simulink model "EVdemo_6"  (R2013b)
settings: Solver=FixedStepDiscrete  SolverMode=SingleTasking  StartTime=0.0  StopTime=650  FixedStep=4e-5  MaxStep=1e-5  RelTol=1e-3
InitFcn:
  | %EV_Param_Update
  | % update the number of strings (discretized)
  | numStrings = round(Opti_numStrings);
  | %disp(['Number of strings: ' num2str(numStrings)])
  | % update the effective capacity based on the number of strings
  | EV_Param.Battery_Det.Rated_Capacity = 28.5*numStrings; %A*hr
  | EV_Param.Battery_Det.DP = 1.5*fliplr([1500 1500 1600 1450 1325 1125 925 675 425 175 ])./8*EV_Param.Battery_Det.Rated_Capacity; % 8 comes from the 8Ahr rated batter data used (normalize and rescale to the rated capacity
  | EV_Param.Battery_Det.CP = fliplr([25 100 200 250 375 550 750 950 1125 1150])./8*EV_Param.Battery_Det.Rated_Capacity;
  | 
  | % update the number of cells in a string (discretized)
  | numSeriesCells = round(Opti_numSeriesCells);
  | %disp(['Number of cells in a string: ' num2str(numSeriesCells)])
  | % update the nominal string volage and charge deficit
  | EV_Param.Battery_Det.Nominal_Voltage = numSeriesCells*cellVolts;
  | BatteryParams(1).Qe_init = 0;%EV_Param.Battery_Det.Rated_Capacity*(1-EV_Param.Battery_Det.Initial_SOC/100); %Ampere*hours
  | 
  | % update the total number of cells, battery pack mass and total vehicle
  | % mass
  | total_cells = numSeriesCells*numStrings;
  | %disp(['Total Number of cells: ' num2str(total_cells)])
  | EV_Param.BatteryMass = BatteryParams(1).cell_mass*total_cells;
  | %disp(['Total Battery Pack Mass: ' num2str(EV_Param.BatteryMass)])
  | EV_Param.Vehicle.Mass = 1300+EV_Param.BatteryMass;
  | 
  | % update the driveline gear ratio
  | EV_Param.Vehicle.Engine_Vehicle_Gear_Ratio = Opti_Vehicle_Gear_Ratio;
  | %disp(['Driveline gear ratio: ' num2str(Opti_Vehicle_Gear_Ratio)])
StartFcn:
  | %tic;
StopFcn:
  | %toc;
  | %disp([Final SOC: ' num2str(SOC_final)])
  | %disp([Final Vehicle Error: ' num2str(normed_SQE_final)])
model workspace (MAT data in the model file):
  MCOS : class17 (value not decoded)
  MCOS : class17 (value not decoded)
values from neighbouring files (symbols this model uses):
  Drive_Cycle_Num = 8    [startDemo.m]
undefined symbols (not defined in the file or in its folder): Acc_Cmd, BatteryParams, Brake_Set, cell_area, ctrlConst, current_phase_a, Dec_Cmd, direct_current, DiscIntNeverNeededParam, electromagnetic_torque, HEV_Param, Ion, Kt_Temps, Lithium, Mech_Power_kW, Opti_numSeriesCells, Opti_numStrings, Opti_Vehicle_Gear_Ratio, paramVelocityI, paramVelocityP, paramVelocityPICurrentSat, pmsm, quadrature_current, RLoadLoss, rotor_velocity, sigbuilder_block, Ts, Veh_Spd_Ref
libraries: fl_lib x306, nesl_utility x100, LeadAcidBattery_lib x60, simulink x23, powerlib x16, sdl_lib x7, elec_lib x4, electricdrivelib x2, checkpacklib x2, CustomDriveline_lib x2, LiBatteryBlocks x1, Capacitors_lib x1
(part 7 of 7)

== system EVdemo_6/Battery/RCGeneric/Measurements/Calculate battery power & charge ==
  -1/(60*60) : fl_lib/Physical Signals/Functions/PS Gain  gain=-1/(60*60)  LocalVarLogging=[]
  Initial charge Ah0 : Integrator  InitialCondition=HEV_Param.Battery_Sys.Maximum_Capacity
  PS Product : fl_lib/Physical Signals/Functions/PS Product  LocalVarLogging=[]
  PS Product1 : fl_lib/Physical Signals/Functions/PS Product  LocalVarLogging=[]
  PS-Simulink Converter : nesl_utility/PS-Simulink Converter  PhysicalDomain=network_engine_domain  SubClassName=ps_output  LeftPortType=input  RightPortType=output  PseudoPeriodic=off  Frequencies=[]  Unit=W  AffineConversion=off
  PS-Simulink Converter1 : nesl_utility/PS-Simulink Converter  PhysicalDomain=network_engine_domain  SubClassName=ps_output  LeftPortType=input  RightPortType=output  PseudoPeriodic=off  Frequencies=[]  Unit=1  AffineConversion=off
  PS-Simulink Converter2 : nesl_utility/PS-Simulink Converter  PhysicalDomain=network_engine_domain  SubClassName=ps_output  LeftPortType=input  RightPortType=output  PseudoPeriodic=off  Frequencies=[]  Unit=1  AffineConversion=off
  Rbat : Gain  Gain=HEV_Param.Battery_Sys.Internal_Resistance
  Terminator : Terminator
  Terminator1 : Terminator
  W to kW : Gain  Gain=1/1000
  V : PMIOPort  Port=1  Side=Left
  I : PMIOPort  Port=2  Side=Left
  Ah : Outport
  wires:
  PS-Simulink Converter/1 -> W to kW/1  "Battery power"
  W to kW/1 -> Terminator/1  "Pe_Batt"
  PS-Simulink Converter1/1 -> Initial charge Ah0/1  "d/dt(Ah)"
  Initial charge Ah0/1 -> Ah/1
  PS-Simulink Converter2/1 -> Rbat/1
  Rbat/1 -> Terminator1/1  "Pr_Batt"
  connections:
  PS Product/RConn1 -- PS-Simulink Converter/LConn1
  V/RConn1 -- PS Product/LConn1
  PS Product/LConn2 -- I/RConn1 -- -1/(60*60)/LConn1 -- PS Product1/LConn1 -- PS Product1/LConn2
  -1/(60*60)/RConn1 -- PS-Simulink Converter1/LConn1
  PS Product1/RConn1 -- PS-Simulink Converter2/LConn1

== system EVdemo_6/DCDC_Converter/Detailed DC//DC Converter/PWM/Sawtooth generator ==
  1\ib3 : Gain  Gain=2  SaturateOnIntegerOverflow=on  OutDataTypeStr=Inherit: Same as input  ParamDataTypeStr=Inherit: Same as input
  Constant1 : Constant  Value=20000
  Constant2 : Constant  Value=2
  Constant3 : Constant
  Discrete-Time Integrator : DiscreteIntegrator  IntegratorMethod=Integration: Trapezoidal  ExternalReset=rising  SampleTime=HEV_Param.DCDCConv.PWM_Carrier_TS  UpperSaturationLimit=1.5  LowerSaturationLimit=-1.5  ICPrevOutput=DiscIntNeverNeededParam  ICPrevScaledInput=DiscIntNeverNeededParam
  Relational Operator1 : RelationalOperator
  Sum1 : Sum  Inputs=+-  SaturateOnIntegerOverflow=on  InputSameDT=on  OutDataTypeStr=Inherit: Same as first input
  Unit Delay : UnitDelay  SampleTime=Ts
  Out : Outport
  wires:
  1\ib3/1 -> Discrete-Time Integrator/1
  Constant3/1 -> Sum1/2
  Sum1/1 -> Out/1
  Unit Delay/1 -> Discrete-Time Integrator/2
  Relational Operator1/1 -> Unit Delay/1
  Constant2/1 -> Relational Operator1/2
  Discrete-Time Integrator/1 -> Sum1/1, Relational Operator1/1
  Constant1/1 -> 1\ib3/1

== system EVdemo_6/DCDC_Converter/Detailed DC//DC Converter/PWM/Thermal Model ==
  IBus : Inport
  1/Mc : Gain  Gain=1/(HEV_Param.DCDCConv.Thermal_Mass*HEV_Param.DCDCConv.Specific_Heat)  SaturateOnIntegerOverflow=on  OutDataTypeStr=Inherit: Same as input  ParamDataTypeStr=Inherit: Same as input
  Air_Temp : Constant  Value=HEV_Param.DCDCConv.Air_Temperature-273
  Heat Losses : Gain  Gain=HEV_Param.DCDCConv.Convection.Area/HEV_Param.DCDCConv.Convection.HT_Coefficient  SaturateOnIntegerOverflow=on  OutDataTypeStr=Inherit: Same as input  ParamDataTypeStr=Inherit: Same as input
  Integrator : Integrator  InitialCondition=HEV_Param.DCDCConv.Initial_Temperature
  Subsystem : Subsystem
  Sum1 : Sum  Inputs=|+-  SaturateOnIntegerOverflow=on  InputSameDT=on  OutDataTypeStr=Inherit: Same as first input
  Sum2 : Sum  Inputs=|+-  SaturateOnIntegerOverflow=on  InputSameDT=on  OutDataTypeStr=Inherit: Same as first input
  tag scope: DCDC_SYS=global
  wires:
  Air_Temp/1 -> Sum2/2
  Subsystem/1(Heat Flow) -> Sum1/1  "Heat In"
  IBus/1 -> Subsystem/1(IBus)
  Integrator/1 -> Sum2/1, [DCDC_SYS]  "DCDC_Temp"
  1/Mc/1 -> Integrator/1
  Heat Losses/1 -> Sum1/2
  Sum2/1 -> Heat Losses/1
  Sum1/1 -> 1/Mc/1

== system EVdemo_6/DCDC_Converter/System DC-DC Converter/Control Bus Voltage/Bus_Control ==
  Err : Inport
  Add : Sum  OutMin=-ctrlConst.CurrentMax*2  OutMax=ctrlConst.CurrentMax*2  OutDataTypeStr=DT_PRECISION_HI  SaturateOnIntegerOverflow=on
      settings: AttributesFormatString=-----------------------------\nMin = %<OutMin>\nMax = %<OutMax>\nSat = %<SaturateOnIntegerOverflow>
  Clamp : Subsystem
  Constant : Constant  Value=0  OutDataTypeStr=Inherit: Inherit via back propagation  PreserveConstantTs=on
  Constant1 : Constant  Value=Ki  SampleTime=-1
  Constant2 : Constant  Value=EV_Param.DCDCConv.PWM_Carrier_TS  OutDataTypeStr=DT_PRECISION_LO  SampleTime=-1
  Convert_Data_Type : Subsystem
      mask Display: fprintf('Double\nRange')
  Maintain_Range : Subsystem
      mask Display: fprintf('Maintain\nRange')
  PI_Sat : Subsystem
      mask Display: plot([0.15 0.85],[.5 .5],[.5 .5],[0.05 0.95],0.15+0.7*[0 .25 .75 1],0.05+0.9*[.25 .25 .75 .75]);
  P_Gain : Gain  Gain=Kp  ParamDataTypeStr=Inherit: Inherit from 'Gain'
      settings: AttributesFormatString=-----------------------------\n%<Gain>
  Product : Product
  Product1 : Product
  Scope1 : Scope
      settings: SaveName=ScopeData13
  Scope2 : Scope
      settings: SaveName=ScopeData14
  Scope3 : Scope
      settings: SaveName=ScopeData15
  Sum : Sum  Inputs=++|
  Switch : Switch  Criteria=u2 > Threshold  InputSameDT=on
  Unit Delay : UnitDelay  SampleTime=-1
  V_Out : Outport
  wires:
  Maintain_Range/1(Out1) -> Product1/2
  Product/1 -> Maintain_Range/1(In1)
  Constant2/1 -> Product/2
  Constant1/1 -> Product/1
  Product1/1 -> Switch/3, Scope3/1, Clamp/3(preIntegrator)
  Clamp/1(Clamp) -> Switch/2
  Constant/1 -> Switch/1
  Unit Delay/1 -> Scope1/1, Sum/2, Add/2  "I_term"
  Add/1 -> Unit Delay/1
  P_Gain/1 -> Convert_Data_Type/1(In1)  "P_term"
  Err/1 -> P_Gain/1, Product1/1
  Switch/1 -> Add/1
  Convert_Data_Type/1(Out1) -> Sum/1, Scope2/1
  PI_Sat/2(saturated) -> Clamp/2(saturated)
  PI_Sat/1(Out1) -> V_Out/1
  Sum/1 -> PI_Sat/1(In1), Clamp/1(preSat)

== system EVdemo_6/Drive & Motor/Detailed_Motor/Motor And Sensors/PMSM_50kW ==
  note: Permanent Magnet
      | Synchronous Machine
  Group Signals : Subsystem
  Measures : electricdrivelib/AC drives/PM Synchronous Motor Drive/Measures
  Mechanical Rotational Reference : fl_lib/Mechanical/Rotational Elements/Mechanical Rotational Reference  t_Log=off  LocalVarNames=|t  LocalVarDescs=|t  LocalVarLogging=0
  Permanent Magnet Synchronous Machine : powerlib/Machines/Permanent Magnet Synchronous Machine  NbPhases=3  FluxDistribution=Sinusoidal  RotorType=Salient-pole  MechanicalLoad=Speed w  PresetModel=No  ShowDetailedParameters=on  Resistance=HEV_Param.Motor.Stator_Resistance  Inductance=8.5e-3  dqInductances=HEV_Param.Motor.Inductances  La=0.000835  MachineConstant=Flux linkage established by magnets (V.s)  Flux=0.175666143629361  VoltageCst=127.4493  TorqueCst=1.054  Flat=120  Mechanical=[0.00062 0.0003035 4 0]  PolePairs=4  InitialConditions=[0,0, 0,0]  InitialConditions5ph=[0 0 0 0 0 0]  TsPowergui=0  TsBlock=-1  RefAngle=Aligned with phase A axis (original Park)
  Rotational Damper : fl_lib/Mechanical/Rotational Elements/Rotational Damper  D=HEV_Param.Motor.Damping N*m/(rad/s)  t_Log=off  w_Log=off  LocalVarNames=|t|w  LocalVarDescs=|t|w  LocalVarLogging=[0 0]
  Shaft Inertia : fl_lib/Mechanical/Rotational Elements/Inertia  inertia=HEV_Param.Motor.Shaft_Inertia kg*m^2  initial_velocity=0 rad/s  t_Log=off  LocalVarNames=|t  LocalVarDescs=|t  LocalVarLogging=0
  Subsystem : Subsystem
      mask Display: disp('GF');
  Subsystem1 : Subsystem
  Terminator : Terminator
  R : PMIOPort  Port=1  Side=Right
  A : PMIOPort  Port=2  Side=Left
  B : PMIOPort  Port=3  Side=Left
  C : PMIOPort  Port=4  Side=Left
  M : Outport
  wires:
  Measures/1 -> Terminator/1
  Permanent Magnet Synchronous Machine/1 -> Subsystem/1(In), Group Signals/1(M)
  Subsystem/1(Out) -> Subsystem1/1(Sig)
  Subsystem1/1(Spd) -> Permanent Magnet Synchronous Machine/1
  Group Signals/1(O) -> M/1  "motor"
  connections:
  C/RConn1 -- Measures/LConn3
  B/RConn1 -- Measures/LConn2
  A/RConn1 -- Measures/LConn1
  Permanent Magnet Synchronous Machine/LConn3 -- Measures/RConn3
  R/RConn1 -- Rotational Damper/LConn1 -- Subsystem1/RConn1 -- Shaft Inertia/LConn1
  Permanent Magnet Synchronous Machine/LConn1 -- Measures/RConn1
  Permanent Magnet Synchronous Machine/LConn2 -- Measures/RConn2
  Mechanical Rotational Reference/LConn1 -- Rotational Damper/RConn1

== system EVdemo_6/Drive & Motor/Detailed_Motor/Motor And Sensors/Temperature Sensor ==
  Ideal Temperature Sensor : fl_lib/Thermal/Thermal Sensors/Ideal Temperature Sensor  Qs_Log=off  Ts_Log=off  LocalVarNames=|Qs|Ts  LocalVarDescs=|Qs|Ts  LocalVarLogging=[]
  PS-Simulink Converter : nesl_utility/PS-Simulink Converter  PhysicalDomain=network_engine_domain  SubClassName=ps_output  LeftPortType=input  RightPortType=output  PseudoPeriodic=off  Frequencies=[]  Unit=C  AffineConversion=on
  Rate Transition5 : RateTransition  OutPortSampleTime=.01
  Thermal Reference : fl_lib/Thermal/Thermal Elements/Thermal Reference  Q_Log=off  LocalVarNames=|Q  LocalVarDescs=|Q  LocalVarLogging=[]
  Conn2 : PMIOPort  Port=1  Side=Left
  tag scope: DCDC_SYS=global
  wires:
  PS-Simulink Converter/1 -> Rate Transition5/1  "DCDC_Temp"
  Rate Transition5/1 -> [DCDC_SYS]
  connections:
  Conn2/RConn1 -- Ideal Temperature Sensor/LConn1
  Thermal Reference/LConn1 -- Ideal Temperature Sensor/RConn1
  PS-Simulink Converter/LConn1 -- Ideal Temperature Sensor/RConn2

== system EVdemo_6/Drive & Motor/System_Motor/Control_Velocity (Explicit_Ts)/Rotor_Velocity_Control ==
  Err : Inport
  mtr_torque_lim : Inport  Port=2  OutMin=-ctrlConst.VelocityMax  OutMax=ctrlConst.VelocityMax
  regen_torque_lim : Inport  Port=3  OutMin=-ctrlConst.VelocityMax  OutMax=ctrlConst.VelocityMax
  Add : Sum  OutMin=-ctrlConst.CurrentMax*2  OutMax=ctrlConst.CurrentMax*2  OutDataTypeStr=DT_PRECISION_HI  SaturateOnIntegerOverflow=on
      settings: AttributesFormatString=-----------------------------\nMin = %<OutMin>\nMax = %<OutMax>\nSat = %<SaturateOnIntegerOverflow>
  Clamp : Subsystem
  Constant : Constant  Value=0  OutDataTypeStr=Inherit: Inherit via back propagation  PreserveConstantTs=on
  Constant1 : Constant  Value=paramVelocityI  SampleTime=-1
  Constant2 : Constant  Value=ctrlConst.Ts  OutDataTypeStr=DT_PRECISION_LO  SampleTime=-1
  Convert_Data_Type : Subsystem
      mask Display: fprintf('Double\nRange')
  Data Type Conversion1 : DataTypeConversion  OutMin=-ctrlConst.CurrentMax  OutMax=ctrlConst.CurrentMax  OutDataTypeStr=DT_PRECISION_LO
      settings: AttributesFormatString=-----------------------------\nMin = %<OutMin>\nMax = %<OutMax>
  Dynamic Saturation : Subsystem
      mask Display: plot([0.15 0.85],[.5 .5],[.5 .5],[0.05 0.95],0.15+0.7*[0 .25 .75 1],0.05+0.9*[.25 .25 .75 .75]);
  Maintain_Range : Subsystem
      mask Display: fprintf('Maintain\nRange')
  PI_Sat1 : Constant  Commented=on  Value=paramVelocityPICurrentSat  PreserveConstantTs=on
  P_Gain : Gain  Gain=paramVelocityP  ParamDataTypeStr=Inherit: Inherit from 'Gain'
      settings: AttributesFormatString=-----------------------------\n%<Gain>
  Product : Product
  Product1 : Product
  Sum : Sum  Inputs=++|
  Switch : Switch  Criteria=u2 > Threshold  InputSameDT=on
  Unit Delay : UnitDelay  SampleTime=-1
  Out : Outport
  wires:
  Data Type Conversion1/1 -> Out/1
  Dynamic Saturation/1(y) -> Data Type Conversion1/1
  Maintain_Range/1(Out1) -> Product1/2
  Product/1 -> Maintain_Range/1(In1)
  Constant2/1 -> Product/2
  Constant1/1 -> Product/1
  Product1/1 -> Switch/3, Clamp/3(preIntegrator)
  Clamp/1(Clamp) -> Switch/2
  Constant/1 -> Switch/1
  Unit Delay/1 -> Sum/2, Add/2  "I_term"
  Add/1 -> Unit Delay/1
  P_Gain/1 -> Convert_Data_Type/1(In1)  "P_term"
  Sum/1 -> Dynamic Saturation/2(u), Clamp/1(preSat)
  Err/1 -> P_Gain/1, Product1/1
  Dynamic Saturation/2(sat_mode) -> Clamp/2(saturated)
  Switch/1 -> Add/1
  Convert_Data_Type/1(Out1) -> Sum/1
  mtr_torque_lim/1 -> Dynamic Saturation/1(up)
  regen_torque_lim/1 -> Dynamic Saturation/3(lo)

== system EVdemo_6/Drive & Motor/System_Motor/Synchronous Motor & Drive/Calculate electrical power ==
  Current Sensor : fl_lib/Electrical/Electrical Sensors/Current Sensor  i1_Log=off  v1_Log=off  LocalVarNames=|i1|v1  LocalVarDescs=|i1|v1  LocalVarLogging=[]
  PS Product1 : fl_lib/Physical Signals/Functions/PS Product  LocalVarLogging=[]
  PS-Simulink Converter : nesl_utility/PS-Simulink Converter  PhysicalDomain=network_engine_domain  SubClassName=ps_output  LeftPortType=input  RightPortType=output  PseudoPeriodic=off  Frequencies=[]  Unit=1  AffineConversion=off
  PS-Simulink Converter1 : nesl_utility/PS-Simulink Converter  PhysicalDomain=network_engine_domain  SubClassName=ps_output  LeftPortType=input  RightPortType=output  PseudoPeriodic=off  Frequencies=[]  Unit=1  AffineConversion=off
  PS-Simulink Converter4 : nesl_utility/PS-Simulink Converter  PhysicalDomain=network_engine_domain  SubClassName=ps_output  LeftPortType=input  RightPortType=output  PseudoPeriodic=off  Frequencies=[]  Unit=1  AffineConversion=off
  Voltage Sensor : fl_lib/Electrical/Electrical Sensors/Voltage Sensor  i1_Log=off  v1_Log=off  LocalVarNames=|i1|v1  LocalVarDescs=|i1|v1  LocalVarLogging=[]
  W to kW : Gain  Gain=1/1000
  + : PMIOPort  Port=1  Side=Left
  ref : PMIOPort  Port=2  Side=Left
  - : PMIOPort  Port=3  Side=Right
  tag scope: Drive_Bus_Current=global, Drive_Bus_Voltage=global, Drive_DC_Power_kW=global
  wires:
  PS-Simulink Converter1/1 -> [Drive_Bus_Current]
  PS-Simulink Converter/1 -> [Drive_Bus_Voltage]
  PS-Simulink Converter4/1 -> W to kW/1
  W to kW/1 -> [Drive_DC_Power_kW]
  connections:
  ref/RConn1 -- Voltage Sensor/RConn2
  +/RConn1 -- Current Sensor/LConn1
  PS-Simulink Converter4/LConn1 -- PS Product1/RConn1
  PS-Simulink Converter/LConn1 -- PS Product1/LConn2 -- Voltage Sensor/RConn1
  Voltage Sensor/LConn1 -- Current Sensor/RConn2 -- -/RConn1
  PS Product1/LConn1 -- PS-Simulink Converter1/LConn1 -- Current Sensor/RConn1

== system EVdemo_6/Drive & Motor/System_Motor/Synchronous Motor & Drive/Calculate mechanical power ==
  Ideal Rotational Motion Sensor : fl_lib/Mechanical/Mechanical Sensors/Ideal Rotational Motion Sensor  offset=0 rad  w_Log=off  t_Log=off  phi_Log=off  LocalVarNames=|w|t|phi  LocalVarDescs=|w|t|phi  LocalVarLogging=[]
  Mechanical Rotational Reference1 : fl_lib/Mechanical/Rotational Elements/Mechanical Rotational Reference  t_Log=off  LocalVarNames=|t  LocalVarDescs=|t  LocalVarLogging=[]
  PS Product : fl_lib/Physical Signals/Functions/PS Product  LocalVarLogging=[]
  PS-Simulink Converter1 : nesl_utility/PS-Simulink Converter  PhysicalDomain=network_engine_domain  SubClassName=ps_output  LeftPortType=input  RightPortType=output  PseudoPeriodic=off  Frequencies=[]  Unit=N*m  AffineConversion=off
  PS-Simulink Converter2 : nesl_utility/PS-Simulink Converter  PhysicalDomain=network_engine_domain  SubClassName=ps_output  LeftPortType=input  RightPortType=output  PseudoPeriodic=off  Frequencies=[]  Unit=rad/s  AffineConversion=off
  PS-Simulink Converter3 : nesl_utility/PS-Simulink Converter  PhysicalDomain=network_engine_domain  SubClassName=ps_output  LeftPortType=input  RightPortType=output  PseudoPeriodic=off  Frequencies=[]  Unit=1  AffineConversion=off
  Torque Sensor : fl_lib/Mechanical/Mechanical Sensors/Ideal Torque Sensor  w_Log=off  t_Log=off  LocalVarNames=|w|t  LocalVarDescs=|w|t  LocalVarLogging=[]
  W to kW : Gain  Gain=1/1000
  C : PMIOPort  Port=1  Side=Right
  R : PMIOPort  Port=2  Side=Left
  tag scope: Motor_Mech_Power_kW=global, Motor_Speed_radps=global, Motor_Torque_Nm=global
  wires:
  PS-Simulink Converter2/1 -> [Motor_Speed_radps]
  W to kW/1 -> [Motor_Mech_Power_kW]
  PS-Simulink Converter3/1 -> W to kW/1
  PS-Simulink Converter1/1 -> [Motor_Torque_Nm]
  connections:
  Mechanical Rotational Reference1/LConn1 -- Ideal Rotational Motion Sensor/RConn1
  PS Product/LConn2 -- PS-Simulink Converter2/LConn1 -- Ideal Rotational Motion Sensor/RConn2
  Torque Sensor/RConn2 -- PS-Simulink Converter1/LConn1 -- PS Product/LConn1
  PS Product/RConn1 -- PS-Simulink Converter3/LConn1
  Ideal Rotational Motion Sensor/LConn1 -- Torque Sensor/LConn1 -- R/RConn1
  C/RConn1 -- Torque Sensor/RConn1

== system EVdemo_6/Drive & Motor/System_Motor/Synchronous Motor & Drive/GF ==
  In1 : Inport
  Simulink-PS Converter : nesl_utility/Simulink-PS Converter  PhysicalDomain=network_engine_domain  SubClassName=ps_input  LeftPortType=input  RightPortType=output  PseudoPeriodic=off  Frequencies=[]  NoiseDistribution=none  NoiseParameters=[]  Unit=1  AffineConversion=off  InputFiltering=off  SimscapeFilterOrder=1  InputFilterTimeConstant=.001  UdotUserProvided=0
  Conn1 : PMIOPort  Port=1  Side=Right
  tag scope: Motor_Torque_Ref=global
  wires:
  In1/1 -> Simulink-PS Converter/1, [Motor_Torque_Ref]
  connections:
  Simulink-PS Converter/RConn1 -- Conn1/RConn1

== system EVdemo_6/Drive & Motor/System_Motor/Synchronous Motor & Drive/PS Terminator1 ==
  PS-Simulink Converter 2 : nesl_utility/PS-Simulink Converter  PhysicalDomain=network_engine_domain  SubClassName=ps_output  LeftPortType=input  RightPortType=output  PseudoPeriodic=off  Frequencies=[]  Unit=rpm  AffineConversion=off
  Terminator : Terminator
  R : PMIOPort  Port=1  Side=Left
  wires:
  PS-Simulink Converter 2/1 -> Terminator/1
  connections:
  R/RConn1 -- PS-Simulink Converter 2/LConn1

== system EVdemo_6/Operator Model/Accel_Cmd_Gen/PI_Sat/Dynamic Saturation ==
  up : Inport
  u : Inport  Port=2
  lo : Inport  Port=3
  Logical Operator : Logic  Operator=OR  AllPortsSameDT=off  OutDataTypeStr=boolean
  LowerRelop1 : RelationalOperator  DisableCoverage=on  Operator=>  OutDataTypeStr=boolean
  Switch : Switch  Criteria=u2 ~= 0  ZeroCross=off
  Switch2 : Switch  Criteria=u2 ~= 0  ZeroCross=off
  UpperRelop : RelationalOperator  DisableCoverage=on  Operator=<  OutDataTypeStr=boolean
  y : Outport
  sat_mode : Outport  Port=2
  wires:
  Logical Operator/1 -> sat_mode/1
  up/1 -> Switch2/1, LowerRelop1/2
  u/1 -> LowerRelop1/1, Switch/3, UpperRelop/1
  lo/1 -> Switch/1, UpperRelop/2
  Switch/1 -> Switch2/3
  Switch2/1 -> y/1
  LowerRelop1/1 -> Switch2/2, Logical Operator/1
  UpperRelop/1 -> Switch/2, Logical Operator/2

== system EVdemo_6/Operator Model/Brake_Cmd_Gen/PI_Sat/Dynamic Saturation ==
  up : Inport
  u : Inport  Port=2
  lo : Inport  Port=3
  Logical Operator : Logic  Operator=OR  AllPortsSameDT=off  OutDataTypeStr=boolean
  LowerRelop1 : RelationalOperator  DisableCoverage=on  Operator=>  OutDataTypeStr=boolean
  Switch : Switch  Criteria=u2 ~= 0  ZeroCross=off
  Switch2 : Switch  Criteria=u2 ~= 0  ZeroCross=off
  UpperRelop : RelationalOperator  DisableCoverage=on  Operator=<  OutDataTypeStr=boolean
  y : Outport
  sat_mode : Outport  Port=2
  wires:
  UpperRelop/1 -> Logical Operator/2, Switch/2
  LowerRelop1/1 -> Logical Operator/1, Switch2/2
  Switch2/1 -> y/1
  Switch/1 -> Switch2/3
  lo/1 -> UpperRelop/2, Switch/1
  u/1 -> UpperRelop/1, Switch/3, LowerRelop1/1
  up/1 -> LowerRelop1/2, Switch2/1
  Logical Operator/1 -> sat_mode/1

== system EVdemo_6/DCDC_Converter/Detailed DC//DC Converter/PWM/Thermal Model/Subsystem ==
  IBus : Inport
  PToHeat : Gain  Gain=HEV_Param.DCDCConv.EPower2Heat  SaturateOnIntegerOverflow=on  OutDataTypeStr=Inherit: Same as input  ParamDataTypeStr=Inherit: Same as input
  Product : Product  RndMeth=Zero
  RLoss : Gain  Gain=HEV_Param.DCDCConv.Resistance_Losses  SaturateOnIntegerOverflow=on  OutDataTypeStr=Inherit: Same as input  ParamDataTypeStr=Inherit: Same as input
  Heat Flow : Outport
  wires:
  PToHeat/1 -> Heat Flow/1
  RLoss/1 -> PToHeat/1
  IBus/1 -> Product/2, Product/1
  Product/1 -> RLoss/1

== system EVdemo_6/DCDC_Converter/System DC-DC Converter/Control Bus Voltage/Bus_Control/Clamp ==
  preSat : Inport
  saturated : Inport  Port=2
  preIntegrator : Inport  Port=3
  AND : Logic  OutDataTypeStr=boolean
  Compare To Zero : simulink/Logic and Bit Operations/Compare To Zero  relop=<=  OutDataTypeStr=boolean
  Compare To Zero1 : simulink/Logic and Bit Operations/Compare To Zero  relop=<=  OutDataTypeStr=boolean
  Logical Operator : Logic  Operator=NXOR  AllPortsSameDT=off  OutDataTypeStr=boolean
  Clamp : Outport
  wires:
  Compare To Zero1/1 -> Logical Operator/2
  Compare To Zero/1 -> Logical Operator/1
  Logical Operator/1 -> AND/1
  preSat/1 -> Compare To Zero1/1
  preIntegrator/1 -> Compare To Zero/1
  saturated/1 -> AND/2
  AND/1 -> Clamp/1

== system EVdemo_6/DCDC_Converter/System DC-DC Converter/Control Bus Voltage/Bus_Control/Convert_Data_Type ==
  In1 : Inport
  Data Type Conversion : DataTypeConversion  Priority=27
  Data Type Propagation : simulink/Signal Attributes/Data Type Propagation  Priority=24  PropDataType=fixdt(1, 16)  IfRefDouble=double  IfRefSingle=single  IsSigned=IsSigned1  NumBitsBase=NumBits1  NumBitsMult=1  NumBitsAdd=0  NumBitsAllowFinal=1:128  PropScaling=2^-10  ValuesUsedBestPrec=[5 -7]  SlopeBase=Slope1  SlopeMult=2  SlopeAdd=0  BiasBase=Bias1  BiasMult=1  BiasAdd=0
      settings: AttributesFormatString=-------------------------------\nDT = %<PropDataType>
  Out1 : Outport
  wires:
  Data Type Conversion/1 -> Data Type Propagation/3, Out1/1
  In1/1 -> Data Type Conversion/1, Data Type Propagation/1, Data Type Propagation/2

== system EVdemo_6/DCDC_Converter/System DC-DC Converter/Control Bus Voltage/Bus_Control/Maintain_Range ==
  In1 : Inport
  Data Type Conversion : DataTypeConversion
  Data Type Propagation : simulink/Signal Attributes/Data Type Propagation  PropDataTypeMode=Specify via dialog  PropDataType=DT_PRECISION_LO  IfRefDouble=double  IfRefSingle=single  IsSigned=IsSigned1  NumBitsBase=NumBits1  NumBitsMult=0  NumBitsAdd=0  NumBitsAllowFinal=1:128  PropScaling=2^-10  ValuesUsedBestPrec=[5 -7]  SlopeBase=PosRange1  SlopeMult=1  SlopeAdd=0  BiasBase=Bias1  BiasMult=1  BiasAdd=0
      settings: AttributesFormatString=-------------------------------\nDT = %<PropDataType>
  Out1 : Outport
  wires:
  Data Type Conversion/1 -> Data Type Propagation/3, Out1/1
  In1/1 -> Data Type Conversion/1, Data Type Propagation/1, Data Type Propagation/2

== system EVdemo_6/DCDC_Converter/System DC-DC Converter/Control Bus Voltage/Bus_Control/PI_Sat ==
  In1 : Inport
  Dynamic Saturation : Subsystem
      mask Display: plot([0.15 0.85],[.5 .5],[.5 .5],[0.05 0.95],0.15+0.7*[0 .25 .75 1],0.05+0.9*[.25 .25 .75 .75]);
  PI_Sat : Constant  Value=800  PreserveConstantTs=on
  PI_Sat1 : Constant  Value=12  PreserveConstantTs=on
  Out1 : Outport
  saturated : Outport  Port=2
  wires:
  In1/1 -> Dynamic Saturation/2(u)
  PI_Sat/1 -> Dynamic Saturation/1(up)
  PI_Sat1/1 -> Dynamic Saturation/3(lo)
  Dynamic Saturation/1(y) -> Out1/1
  Dynamic Saturation/2(sat_mode) -> saturated/1

== system EVdemo_6/Drive & Motor/Detailed_Motor/Motor And Sensors/PMSM_50kW/Group Signals ==
  note: Group Signals
  note: Rename signals provided to output bus.
  M : Inport
  Bus Creator2 : BusCreator  Inputs=10
  Bus Selector2 : BusSelector  OutputSignals=Stator current is_a (A),Stator current is_b (A),Stator current is_c (A),Electromagnetic torque Te (N*m),Rotor speed wm (rad/s),Stator current is_d (A),Stator current is_q (A),Rotor angle thetam (rad)
  Mechanical To Electrical : Subsystem
  Signal Conversion {1..5,7..8} (7 alike) : SignalConversion  ConversionOutput=Contiguous copy
  Wrap 2pi : Subsystem
  O : Outport
  wires:
  Bus Creator2/1 -> O/1  "measure"
  M/1 -> Bus Selector2/1, Mechanical To Electrical/1(M)
  Bus Selector2/1 -> Signal Conversion 1/1  "<Stator current is_a (A)>"
  Bus Selector2/2 -> Signal Conversion 2/1  "<Stator current is_b (A)>"
  Bus Selector2/3 -> Signal Conversion 3/1  "<Stator current is_c (A)>"
  Bus Selector2/5 -> Signal Conversion 5/1  "<Rotor speed wm (rad/s)>"
  Bus Selector2/4 -> Signal Conversion 4/1  "<Electromagnetic torque Te (N*m)>"
  Signal Conversion 1/1 -> Bus Creator2/1  "current_phase_a"
  Signal Conversion 2/1 -> Bus Creator2/2  "current_phase_b"
  Signal Conversion 3/1 -> Bus Creator2/3  "current_phase_c"
  Signal Conversion 4/1 -> Bus Creator2/4  "electromagnetic_torque"
  Signal Conversion 5/1 -> Bus Creator2/5  "rotor_velocity"
  Bus Selector2/8 -> Wrap 2pi/1(M)  "<Rotor angle thetam (rad)>"
  Signal Conversion 7/1 -> Bus Creator2/6  "direct_current"
  Signal Conversion 8/1 -> Bus Creator2/7  "quadrature_current"
  Bus Selector2/6 -> Signal Conversion 7/1  "<Stator current is_d (A)>"
  Bus Selector2/7 -> Signal Conversion 8/1  "<Stator current is_q (A)>"
  Wrap 2pi/1(Position) -> Bus Creator2/8  "rotor_position"
  Mechanical To Electrical/1(Position) -> Bus Creator2/9  "electrical_position"
  Mechanical To Electrical/2(Velocity) -> Bus Creator2/10  "electrical_velocity"

== system EVdemo_6/Drive & Motor/Detailed_Motor/Motor And Sensors/PMSM_50kW/Subsystem ==
  In : Inport
  "+ -> -1" : Gain  Gain=30/pi
  Bus Selector : BusSelector  OutputSignals=Stator current is_a (A),Rotor speed wm (rad/s),Electromagnetic torque Te (N*m)
  Mux1 : Mux  Inputs=2
  Mux2 : Mux  Inputs=3
  Out : Outport
  tag scope: MotorDrive=global
  wires:
  In/1 -> Bus Selector/1, Out/1
  "+ -> -1"/1 -> Mux2/2
  [Mot_TReq_SYS] -> Mux1/2
  Bus Selector/2 -> "+ -> -1"/1  "<Rotor speed wm (rad/s)>"
  Bus Selector/3 -> Mux1/1  "<Electromagnetic torque Te (N*m)>"
  Mux1/1 -> Mux2/3
  Bus Selector/1 -> Mux2/1  "<Stator current is_a (A)>"
  Mux2/1 -> [MotorDrive]

== system EVdemo_6/Drive & Motor/Detailed_Motor/Motor And Sensors/PMSM_50kW/Subsystem1 ==
  Sig : Inport
  Bus Selector : BusSelector  OutputSignals=Electromagnetic torque Te (N*m)
  Ideal Rotational Motion Sensor : fl_lib/Mechanical/Mechanical Sensors/Ideal Rotational Motion Sensor  offset=0 rad  w_Log=off  t_Log=off  phi_Log=off  LocalVarNames=|w|t|phi  LocalVarDescs=|w|t|phi  LocalVarLogging=[0 0 0]
  Ideal Torque Source : fl_lib/Mechanical/Mechanical Sources/Ideal Torque Source  w_Log=off  t_Log=off  LocalVarNames=|w|t  LocalVarDescs=|w|t  LocalVarLogging=[0 0]
  Mechanical Rotational Reference : fl_lib/Mechanical/Rotational Elements/Mechanical Rotational Reference  t_Log=off  LocalVarNames=|t  LocalVarDescs=|t  LocalVarLogging=0
  Mechanical Rotational Reference1 : fl_lib/Mechanical/Rotational Elements/Mechanical Rotational Reference  t_Log=off  LocalVarNames=|t  LocalVarDescs=|t  LocalVarLogging=0
  PS-Simulink Converter : nesl_utility/PS-Simulink Converter  PhysicalDomain=network_engine_domain  SubClassName=ps_output  LeftPortType=input  RightPortType=output  PseudoPeriodic=off  Frequencies=[]  Unit=rad/s  AffineConversion=off
  Rate Transition : RateTransition
  Rate Transition1 : RateTransition
  Simulink-PS Converter : nesl_utility/Simulink-PS Converter  PhysicalDomain=network_engine_domain  SubClassName=ps_input  LeftPortType=input  RightPortType=output  PseudoPeriodic=off  Frequencies=[]  NoiseDistribution=none  NoiseParameters=[]  Unit=1  AffineConversion=off  InputFiltering=off  SimscapeFilterOrder=1  InputFilterTimeConstant=.001  UdotUserProvided=0
  Sh : PMIOPort  Port=1  Side=Right
  Spd : Outport
  tag scope: MotorTorque_Nm=global
  wires:
  PS-Simulink Converter/1 -> Rate Transition/1
  Sig/1 -> Bus Selector/1
  Bus Selector/1 -> [MotorTorque_Nm], Rate Transition1/1  "<Electromagnetic torque Te (N*m)>"
  Rate Transition/1 -> Spd/1
  Rate Transition1/1 -> Simulink-PS Converter/1
  connections:
  Simulink-PS Converter/RConn1 -- Ideal Torque Source/RConn1
  PS-Simulink Converter/LConn1 -- Ideal Rotational Motion Sensor/RConn2
  Ideal Rotational Motion Sensor/LConn1 -- Sh/RConn1 -- Ideal Torque Source/LConn1
  Mechanical Rotational Reference1/LConn1 -- Ideal Torque Source/RConn2
  Mechanical Rotational Reference/LConn1 -- Ideal Rotational Motion Sensor/RConn1

== system EVdemo_6/Drive & Motor/System_Motor/Control_Velocity (Explicit_Ts)/Rotor_Velocity_Control/Clamp ==
  preSat : Inport
  saturated : Inport  Port=2
  preIntegrator : Inport  Port=3
  AND : Logic  OutDataTypeStr=boolean
  Compare To Zero : simulink/Logic and Bit Operations/Compare To Zero  relop=<=  OutDataTypeStr=boolean
  Compare To Zero1 : simulink/Logic and Bit Operations/Compare To Zero  relop=<=  OutDataTypeStr=boolean
  Logical Operator : Logic  Operator=NXOR  AllPortsSameDT=off  OutDataTypeStr=boolean
  Clamp : Outport
  wires:
  Compare To Zero1/1 -> Logical Operator/2
  Compare To Zero/1 -> Logical Operator/1
  Logical Operator/1 -> AND/1
  preSat/1 -> Compare To Zero1/1
  preIntegrator/1 -> Compare To Zero/1
  saturated/1 -> AND/2
  AND/1 -> Clamp/1

== system EVdemo_6/Drive & Motor/System_Motor/Control_Velocity (Explicit_Ts)/Rotor_Velocity_Control/Convert_Data_Type ==
  In1 : Inport
  Data Type Conversion : DataTypeConversion  Priority=27
  Data Type Propagation : simulink/Signal Attributes/Data Type Propagation  Priority=24  PropDataType=fixdt(1, 16)  IfRefDouble=double  IfRefSingle=single  IsSigned=IsSigned1  NumBitsBase=NumBits1  NumBitsMult=1  NumBitsAdd=0  NumBitsAllowFinal=1:128  PropScaling=2^-10  ValuesUsedBestPrec=[5 -7]  SlopeBase=Slope1  SlopeMult=2  SlopeAdd=0  BiasBase=Bias1  BiasMult=1  BiasAdd=0
      settings: AttributesFormatString=-------------------------------\nDT = %<PropDataType>
  Out1 : Outport
  wires:
  Data Type Conversion/1 -> Data Type Propagation/3, Out1/1
  In1/1 -> Data Type Conversion/1, Data Type Propagation/1, Data Type Propagation/2

== system EVdemo_6/Drive & Motor/System_Motor/Control_Velocity (Explicit_Ts)/Rotor_Velocity_Control/Dynamic Saturation ==
  up : Inport
  u : Inport  Port=2
  lo : Inport  Port=3
  Logical Operator : Logic  Operator=OR  AllPortsSameDT=off  OutDataTypeStr=boolean
  LowerRelop1 : RelationalOperator  DisableCoverage=on  Operator=>  OutDataTypeStr=boolean
  Switch : Switch  Criteria=u2 ~= 0  ZeroCross=off
  Switch2 : Switch  Criteria=u2 ~= 0  ZeroCross=off
  UpperRelop : RelationalOperator  DisableCoverage=on  Operator=<  OutDataTypeStr=boolean
  y : Outport
  sat_mode : Outport  Port=2
  wires:
  UpperRelop/1 -> Logical Operator/2, Switch/2
  LowerRelop1/1 -> Logical Operator/1, Switch2/2
  Switch2/1 -> y/1
  Switch/1 -> Switch2/3
  lo/1 -> UpperRelop/2, Switch/1
  u/1 -> UpperRelop/1, Switch/3, LowerRelop1/1
  up/1 -> LowerRelop1/2, Switch2/1
  Logical Operator/1 -> sat_mode/1

== system EVdemo_6/Drive & Motor/System_Motor/Control_Velocity (Explicit_Ts)/Rotor_Velocity_Control/Maintain_Range ==
  In1 : Inport
  Data Type Conversion : DataTypeConversion
  Data Type Propagation : simulink/Signal Attributes/Data Type Propagation  PropDataTypeMode=Specify via dialog  PropDataType=DT_PRECISION_LO  IfRefDouble=double  IfRefSingle=single  IsSigned=IsSigned1  NumBitsBase=NumBits1  NumBitsMult=0  NumBitsAdd=0  NumBitsAllowFinal=1:128  PropScaling=2^-10  ValuesUsedBestPrec=[5 -7]  SlopeBase=PosRange1  SlopeMult=1  SlopeAdd=0  BiasBase=Bias1  BiasMult=1  BiasAdd=0
      settings: AttributesFormatString=-------------------------------\nDT = %<PropDataType>
  Out1 : Outport
  wires:
  Data Type Conversion/1 -> Data Type Propagation/3, Out1/1
  In1/1 -> Data Type Conversion/1, Data Type Propagation/1, Data Type Propagation/2

== system EVdemo_6/DCDC_Converter/System DC-DC Converter/Control Bus Voltage/Bus_Control/PI_Sat/Dynamic Saturation ==
  up : Inport
  u : Inport  Port=2
  lo : Inport  Port=3
  Logical Operator : Logic  Operator=OR  AllPortsSameDT=off  OutDataTypeStr=boolean
  LowerRelop1 : RelationalOperator  DisableCoverage=on  Operator=>  OutDataTypeStr=boolean
  Switch : Switch  Criteria=u2 ~= 0  ZeroCross=off
  Switch2 : Switch  Criteria=u2 ~= 0  ZeroCross=off
  UpperRelop : RelationalOperator  DisableCoverage=on  Operator=<  OutDataTypeStr=boolean
  y : Outport
  sat_mode : Outport  Port=2
  wires:
  UpperRelop/1 -> Logical Operator/2, Switch/2
  LowerRelop1/1 -> Logical Operator/1, Switch2/2
  Switch2/1 -> y/1
  Switch/1 -> Switch2/3
  lo/1 -> UpperRelop/2, Switch/1
  u/1 -> UpperRelop/1, Switch/3, LowerRelop1/1
  up/1 -> LowerRelop1/2, Switch2/1
  Logical Operator/1 -> sat_mode/1

== system EVdemo_6/Drive & Motor/Detailed_Motor/Motor And Sensors/PMSM_50kW/Group Signals/Mechanical To Electrical ==
  M : Inport
  Bus Selector1 : BusSelector  OutputSignals=Rotor angle thetam (rad)
  Bus Selector2 : BusSelector  OutputSignals=Rotor speed wm (rad/s)
  Gain1 : Gain  Gain=pmsm.PolePairs
      settings: AttributesFormatString=-----------------------------\n%<Gain>
  Gain2 : Gain  Gain=pmsm.PolePairs
      settings: AttributesFormatString=-----------------------------\n%<Gain>
  Modulus : Math  Operator=mod  SaturateOnIntegerOverflow=on
  Two Pi : Constant  Value=2*pi  OutDataTypeStr=Inherit: Inherit via back propagation
  Position : Outport
  Velocity : Outport  Port=2
  wires:
  M/1 -> Bus Selector1/1, Bus Selector2/1
  Two Pi/1 -> Modulus/2
  Bus Selector1/1 -> Gain1/1  "<Rotor angle thetam (rad)>"
  Modulus/1 -> Position/1
  Gain1/1 -> Modulus/1
  Bus Selector2/1 -> Gain2/1  "<Rotor speed wm (rad/s)>"
  Gain2/1 -> Velocity/1

== system EVdemo_6/Drive & Motor/Detailed_Motor/Motor And Sensors/PMSM_50kW/Group Signals/Wrap 2pi ==
  M : Inport
  Modulus : Math  Operator=mod  SaturateOnIntegerOverflow=on
  Two Pi : Constant  Value=2*pi  OutDataTypeStr=Inherit: Inherit via back propagation
  Position : Outport
  wires:
  Two Pi/1 -> Modulus/2
  Modulus/1 -> Position/1
  M/1 -> Modulus/1

== stateflow chart EVdemo_6/Operator Model/Chart ==
  state Stop
    du: Mode=0;
    du: BrakeSet = 1;
  state Accel
    du: Mode=1;
  state Decel
    du: Mode = 2;
  (default) -> Stop
  (junction 32) -> Stop
  Decel -> (junction 32) [order 2] : [Spd_Ref <=0 && veh_spd<0.125]
  Stop -> Accel : [(spd_err>0.25)]
      | {BrakeSet=0;}
  Accel -> Decel : [(spd_err<-1) &&(spd_ref_rate<0 || spd_err<-3) && after(10,tick)]
  Decel -> Accel [order 1] : [(spd_err>1 ) && (spd_ref_rate>0 || spd_err>3) && after(10,tick)]
  data: Spd_Ref input; Mode output uint8 =0; spd_err input; veh_spd input; BrakeSet output boolean; spd_ref_rate input
